simulink model "pi_model"  (R2016b)
settings: Solver=VariableStepAuto  StartTime=0.0  StopTime=10.0  RelTol=1e-3
undefined symbols (not defined in the file or in its folder): Params
settings Model: Creator=sembl  LastModifiedBy=sembl

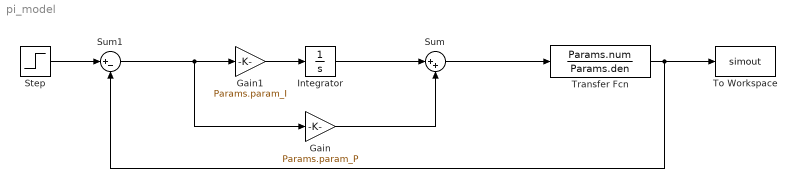
== system pi_model ==
  Gain : Gain  Gain=Params.param_P
  Gain1 : Gain  Gain=Params.param_I
  Integrator : Integrator
  Step : Step  Time=5  Before=1  After=0  SampleTime=0
  Sum : Sum  Inputs=|++
  Sum1 : Sum  Inputs=|+-
  To Workspace : ToWorkspace  VariableName=simout  SaveFormat=Timeseries  SampleTime=-1
  Transfer Fcn : TransferFcn  Numerator=Params.num  Denominator=Params.den
  wires:
  Integrator/1 -> Sum/1
  Gain/1 -> Sum/2
  Sum/1 -> Transfer Fcn/1
  Gain1/1 -> Integrator/1
  Sum1/1 -> Gain/1, Gain1/1
  Transfer Fcn/1 -> To Workspace/1, Sum1/2
  Step/1 -> Sum1/1
